simulink model "quy_dao_3diem_5lan"  (R2022b)
settings: Solver=FixedStepAuto  StartTime=0.0  StopTime=30  FixedStep=0.01  RelTol=1e-3
settings Model: Creator=Admin  LastModifiedBy=Admin

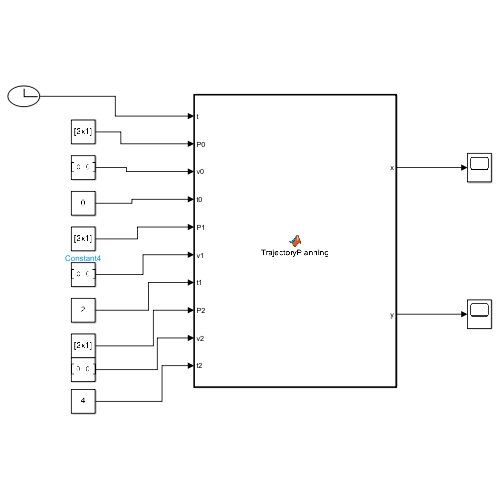
[thumbnail: Simulink's stored preview of the top-level diagram]
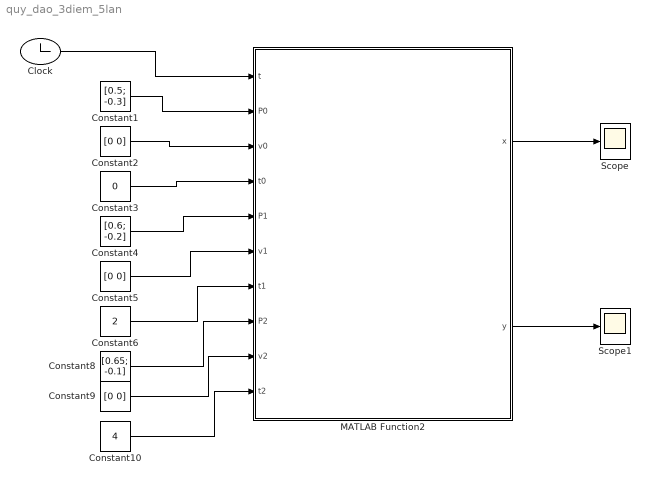
== system quy_dao_3diem_5lan ==
  Clock : Clock
      settings: Decimation=20
  Constant1 : Constant  Value=[0.5; -0.3]
  Constant10 : Constant  Value=4
  Constant2 : Constant  Value=[0 0]
  Constant3 : Constant  Value=0
  Constant4 : Constant  Value=[0.6; -0.2]
  Constant5 : Constant  Value=[0 0]
  Constant6 : Constant  Value=2
  Constant8 : Constant  Value=[0.65; -0.1]
  Constant9 : Constant  Value=[0 0]
  MATLAB Function2 : MATLAB Function  TreatAsAtomicUnit=on
  Scope : Scope
  Scope1 : Scope
  wires:
  Constant6/1 -> MATLAB Function2/7(t1)
  Constant2/1 -> MATLAB Function2/3(v0)
  Clock/1 -> MATLAB Function2/1(t)
  Constant3/1 -> MATLAB Function2/4(t0)
  MATLAB Function2/1(x) -> Scope/1
  Constant5/1 -> MATLAB Function2/6(v1)
  Constant1/1 -> MATLAB Function2/2(P0)
  Constant4/1 -> MATLAB Function2/5(P1)
  Constant8/1 -> MATLAB Function2/8(P2)
  Constant9/1 -> MATLAB Function2/9(v2)
  Constant10/1 -> MATLAB Function2/10(t2)
  MATLAB Function2/2(y) -> Scope1/1

== matlab function quy_dao_3diem_5lan/MATLAB Function2 ==
  data: t input; x output; y output; P0 input; v0 input; t0 input; P1 input; v1 input; t1 input; P2 input; v2 input; t2 input
function [x,y] = TrajectoryPlanning(t,P0,v0,t0,P1,v1,t1,P2,v2,t2)
a10_AB=P0(1);
a20_AB=P0(2);
a11_AB=v0(1);
a21_AB=v0(2);
a12_AB=3/(t1-t0)^2*(P1(1)-P0(1))-2/(t1-t0)*v0(1)-1/(t1-t0)*v1(1);
a22_AB=3/(t1-t0)^2*(P1(2)-P0(2))-2/(t1-t0)*v0(2)-1/(t1-t0)*v1(2);
a13_AB=-2/(t1-t0)^3*(P1(1)-P0(1))+1/(t1-t0)^2*(v1(1)+v0(1));
a23_AB=-2/(t1-t0)^3*(P1(2)-P0(2))+1/(t1-t0)^2*(v1(2)+v0(2));

a10_BC=P1(1);
a20_BC=P1(2);
a11_BC=v1(1);
a21_BC=v1(2);
a12_BC=3/(t2-t1)^2*(P2(1)-P1(1))-2/(t2-t1)*v1(1)-1/(t2-t1)*v2(1);
a22_BC=3/(t2-t1)^2*(P2(2)-P1(2))-2/(t2-t1)*v1(2)-1/(t2-t1)*v2(2);
a13_BC=-2/(t2-t1)^3*(P2(1)-P1(1))+1/(t2-t1)^2*(v2(1)+v1(1));
a23_BC=-2/(t2-t1)^3*(P2(2)-P1(2))+1/(t2-t1)^2*(v2(2)+v1(2));

a10_CA=P2(1);
a20_CA=P2(2);
a11_CA=v2(1);
a21_CA=v2(2);
a12_CA=3/(t0-t2)^2*(P0(1)-P2(1))-2/(t0-t2)*v2(1)-1/(t0-t2)*v0(1);
a22_CA=3/(t0-t2)^2*(P0(2)-P2(2))-2/(t0-t2)*v2(2)-1/(t0-t2)*v0(2);
a13_CA=-2/(t0-t2)^3*(P0(1)-P2(1))+1/(t0-t2)^2*(v0(1)+v2(1));
a23_CA=-2/(t0-t2)^3*(P0(2)-P2(2))+1/(t0-t2)^2*(v0(2)+v2(2));

i=fix(t/t1)+1;
k = fix(t/6)+1;

if (i == 1 + (k-1)*3)
      tt=t-2*(i-1);
      x=a10_AB+a11_AB*tt+a12_AB*tt^2+a13_AB*tt^3;
      y=a20_AB+a21_AB*tt+a22_AB*tt^2+a23_AB*tt^3;
elseif (i == 2 + (k-1)*3)
      tt=t-2*(i-1);
      x=a10_BC+a11_BC*tt+a12_BC*tt^2+a13_BC*tt^3;
      y=a20_BC+a21_BC*tt+a22_BC*tt^2+a23_BC*tt^3;
elseif(i == 3 + (k-1)*3)
      tt=t-2*(i-1);
      x=a10_CA+a11_CA*tt+a12_CA*tt^2+a13_CA*tt^3;
      y=a20_CA+a21_CA*tt+a22_CA*tt^2+a23_CA*tt^3;
else
      x=P0(1);
      y=P0(2);
end
